simulink model "EKF"  (R2024b)
settings: Solver=ode4  StartTime=0.0  StopTime=10  FixedStep=1e-2  RelTol=1e-3
values from neighbouring files (symbols this model uses):
  L = 10e-2    (= 0.1)    [EKF.m]
  Q = eye(8)*0.1    [EKF.m]
  R = eye(2)*10    [EKF.m]
  r = 3.5e-2    (= 0.035)    [EKF.m]
  theta_0 = deg2rad(0)    [EKF.m]
  Ts = 1/10    (= 0.1)    [EKF.m]
libraries: simulink x5, sharedTrackingLibrary x1
settings Model: ParamWorkspaceSource=ReferencedWorkspace  Creator=pedro  LastModifiedBy=pedro
settings SFSimCC: SimCustomHeaderCode="#include \"EstimationSystem.h\""  SimUserSources=C:\Users\pedro\Documents\UNICAMP\embarcados\ekf_cross_plat\src\EstimationSystem.c  SimUserLibraries=C:\Users\pedro\Documents\UNICAMP\embarcados\ekf_cross_plat\build\lib\CMSIS-DSP\Source\libCMSISDSP.a  SimCustomCompilerFlags=-DARM_MATH_LOOPUNROLL -D__GNUC_PYTHON__  CustomCodeGlobalsAsFunctionIO=on  SimHardwareAcceleration=off
settings SFSimCC: SimUserIncludeDirs=|
  | C:\Users\pedro\Documents\UNICAMP\embarcados\ekf_cross_plat\inc
  | C:\Users\pedro\Documents\UNICAMP\embarcados\ekf_cross_plat\lib\CMSIS-DSP\Include
  | C:\Users\pedro\Documents\UNICAMP\embarcados\ekf_cross_plat\lib\CMSIS-DSP\PrivateInclude
  | C:\Users\pedro\Documents\UNICAMP\embarcados\ekf_cross_plat\lib\CMSIS-DSP\Source\DistanceFunctions
  | C:\Users\pedro\Documents\UNICAMP\embarcados\ekf_cross_plat\lib\CMSIS-DSP\ComputeLibrary
settings RTWCC: GenerateReport=on  RTWUseSimCustomCode=on  CustomHeaderCode="#include \"EstimationSystem.h\""  CustomSource=C:\Users\pedro\Documents\UNICAMP\embarcados\ekf_cross_plat\src\EstimationSystem.c  CustomLibrary=C:\Users\pedro\Documents\UNICAMP\embarcados\ekf_cross_plat\build\lib\CMSIS-DSP\Source\libCMSISDSP.a  BuildConfiguration=Debug  LaunchReport=on
settings RTWCC: CustomInclude=|
  | C:\Users\pedro\Documents\UNICAMP\embarcados\ekf_cross_plat\inc
  | C:\Users\pedro\Documents\UNICAMP\embarcados\ekf_cross_plat\lib\CMSIS-DSP\Include
  | C:\Users\pedro\Documents\UNICAMP\embarcados\ekf_cross_plat\lib\CMSIS-DSP\PrivateInclude
  | C:\Users\pedro\Documents\UNICAMP\embarcados\ekf_cross_plat\lib\CMSIS-DSP\Source\DistanceFunctions
  | C:\Users\pedro\Documents\UNICAMP\embarcados\ekf_cross_plat\lib\CMSIS-DSP\ComputeLibrary
settings CodeAppCC: MaxIdLength=95

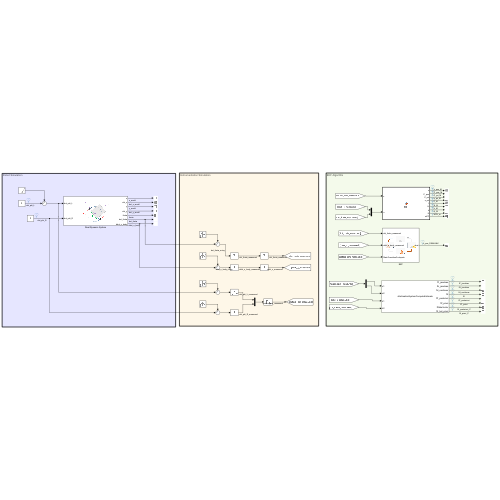
[thumbnail: Simulink's stored preview of the top-level diagram]
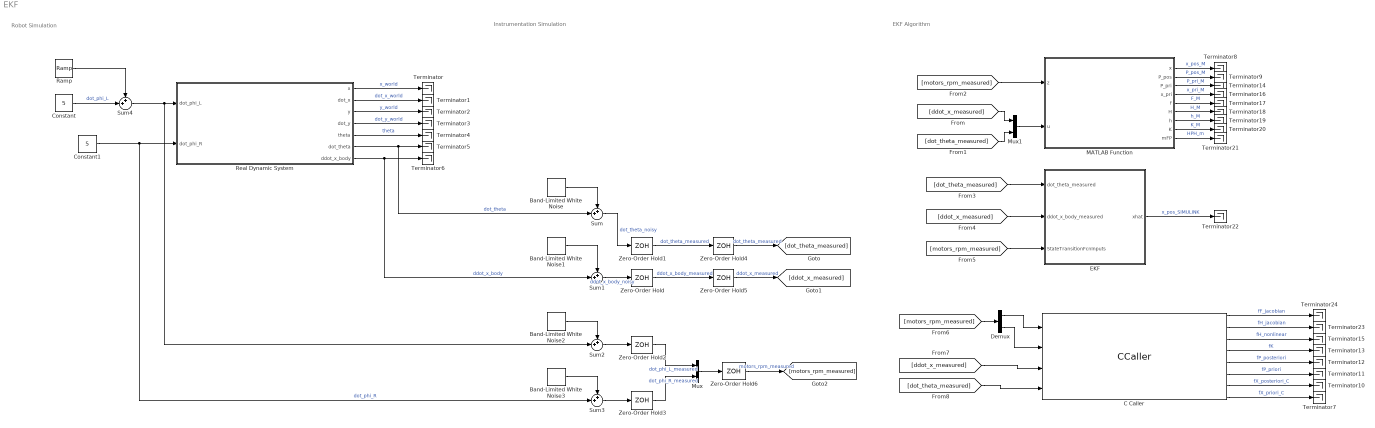
== system EKF ==
  note: EKF Algorithm
  note: Instrumentation Simulation
  note: Robot Simulation
  Band-Limited White Noise : simulink/Sources/Band-Limited White Noise  Cov=[0.0001]  Ts=0.1  seed=[23341]
  Band-Limited White Noise1 : simulink/Sources/Band-Limited White Noise  Cov=[0.0001]  Ts=0.1  seed=[23341]
  Band-Limited White Noise2 : simulink/Sources/Band-Limited White Noise  Cov=[0.001]  Ts=0.1  seed=[23341]
  Band-Limited White Noise3 : simulink/Sources/Band-Limited White Noise  Cov=[0.001]  Ts=0.1  seed=[23341]
  C Caller : CCaller  FunctionName=vEstimationSystemComputeEstimate  PortSpecificationStruct="%)30     .     !4   8    (     @         %    \"     P    !     0         %  0 \"0    $    _    07)G3F%M90  4&]R=$YA;64 4V-O<&4     26YD97@     5'EP90      4VEZ90      27-';&]B86P   X    P    !@    @    $          4    (     0    (    !         !   @!U,0  #@   #     &    \"     0         !0    @    !     @    $         $  \" '4Q   .    .     8    (    !          %    \"     $    %     0         0  ...(+6883 chars)"  SampleTime=Ts
  Constant : Constant  Value=5
  Constant1 : Constant  Value=5
  Demux : Demux  Outputs=2
  EKF : Subsystem
      mask Display: image('EKF_icon.png', [0,0,0,0,90,90]);
  MATLAB Function : MATLAB Function  TreatAsAtomicUnit=on
  Mux : Mux  Inputs=2
  Mux1 : Mux  Inputs=2
  Ramp : simulink/Sources/Ramp  slope=1  start=2  InitialOutput=0
  Real Dynamic System : Subsystem
      mask Display: image('robot_model.png', [0,0,0,0,90,90]);
  Sum{,1..4} (5 alike) : Sum  Inputs=++|
  Terminator{,1..24} (25 alike) : Terminator
  Zero-Order Hold{,1..6} (7 alike) : ZeroOrderHold  SampleTime=Ts
  wires:
  Constant/1 -> Sum4/2  "dot_phi_L"
  Constant1/1 -> Real Dynamic System/2(dot_phi_R), Sum3/2  "dot_phi_R"
  Real Dynamic System/1(x) -> Terminator/1  "x_world"
  Real Dynamic System/2(dot_x) -> Terminator1/1  "dot_x_world"
  Real Dynamic System/3(y) -> Terminator2/1  "y_world"
  Real Dynamic System/4(dot_y) -> Terminator3/1  "dot_y_world"
  Real Dynamic System/5(theta) -> Terminator4/1  "theta"
  Real Dynamic System/6(dot_theta) -> Sum/2, Terminator5/1  "dot_theta"
  Real Dynamic System/7(ddot_x_body) -> Sum1/2, Terminator6/1  "ddot_x_body"
  Band-Limited White Noise/1 -> Sum/1
  Sum/1 -> Zero-Order Hold1/1  "dot_theta_noisy"
  Band-Limited White Noise1/1 -> Sum1/1
  Sum1/1 -> Zero-Order Hold/1  "ddot_x_body_noisy"
  Band-Limited White Noise2/1 -> Sum2/1
  Band-Limited White Noise3/1 -> Sum3/1
  Sum2/1 -> Zero-Order Hold2/1
  Sum3/1 -> Zero-Order Hold3/1
  Mux/1 -> Zero-Order Hold6/1
  Zero-Order Hold1/1 -> Zero-Order Hold4/1  "dot_theta_measured"
  Zero-Order Hold/1 -> Zero-Order Hold5/1  "ddot_x_body_measured"
  Zero-Order Hold2/1 -> Mux/1  "dot_phi_L_measured"
  Zero-Order Hold3/1 -> Mux/2  "dot_phi_R_measured"
  Zero-Order Hold4/1 -> [dot_theta_measured]  "dot_theta_measured"
  Zero-Order Hold5/1 -> [ddot_x_measured]  "ddot_x_measured"
  Zero-Order Hold6/1 -> [motors_rpm_measured]  "motors_rpm_measured"
  Sum4/1 -> Sum2/2, Real Dynamic System/1(dot_phi_L)
  Ramp/1 -> Sum4/1
  MATLAB Function/1(x) -> Terminator8/1  "x_pos_M"
  [ddot_x_measured] -> Mux1/1
  [dot_theta_measured] -> Mux1/2
  [dot_theta_measured] -> EKF/1(dot_theta_measured)
  [ddot_x_measured] -> EKF/2(ddot_x_body_measured)
  [motors_rpm_measured] -> EKF/3(StateTransitionFcnInputs)
  [motors_rpm_measured] -> Demux/1
  Demux/1 -> C Caller/1
  Demux/2 -> C Caller/2
  [ddot_x_measured] -> C Caller/3
  [dot_theta_measured] -> C Caller/4
  Mux1/1 -> MATLAB Function/2(u)
  [motors_rpm_measured] -> MATLAB Function/1(z)
  MATLAB Function/2(P_pos) -> Terminator9/1  "P_pos_M"
  MATLAB Function/3(P_pri) -> Terminator14/1  "P_pri_M"
  MATLAB Function/4(x_pri) -> Terminator16/1  "x_pri_M"
  MATLAB Function/5(f) -> Terminator17/1  "F_M"
  MATLAB Function/6(H) -> Terminator18/1  "H_M"
  MATLAB Function/7(h) -> Terminator19/1  "h_M"
  MATLAB Function/8(K) -> Terminator20/1  "K_M"
  MATLAB Function/9(mFP) -> Terminator21/1  "HPH_m"
  EKF/1(xhat) -> Terminator22/1  "x_pos_SIMULINK"
  C Caller/8 -> Terminator7/1  "fX_priori_C"
  C Caller/7 -> Terminator10/1  "fX_posteriori_C"
  C Caller/6 -> Terminator11/1  "fP_priori"
  C Caller/5 -> Terminator12/1  "fP_posteriori"
  C Caller/4 -> Terminator13/1  "fK"
  C Caller/3 -> Terminator15/1  "fH_nonlinear"
  C Caller/2 -> Terminator23/1  "fH_jacobian"
  C Caller/1 -> Terminator24/1  "fF_jacobian"

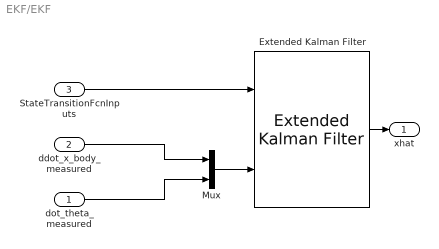
== system EKF/EKF ==
  dot_theta_measured : Inport
  ddot_x_body_measured : Inport  Port=2
  StateTransitionFcnInputs : Inport  Port=3
  Extended Kalman Filter : sharedTrackingLibrary/Extended Kalman Filter  StateTransitionFcn=DifferentialRobotModel  HasStateTransitionJacobianFcn=on  StateTransitionJacobianFcn=A_Jacobian  HasAdditiveProcessNoise=Additive  ProcessNoise=eye(8)*0.1  HasTimeVaryingProcessNoise=off  HasStateTransitionFcnExtraArgument=1  InitialState=states_0  InitialStateCovariance=eye(8)*0.1  MeasurementFcn1=OBSERVATION_h  HasMeasurementJacobianFcn1=on  MeasurementJacobianFcn1=H_jacobian  HasMeasurementEnablePort1=off  HasAdditiveMeasurementNoise1=Additive  MeasurementNoise1=eye(2)*10  HasTimeVaryingMeasurementNoise1=off  HasMeasurementFcnExtraArgument1=0  HasMeasurementWrapping1=off  MeasurementFcn2=OBSERVATION_x_ddot_body  HasMeasurementJacobianFcn2=off  HasMeasurementEnablePort2=off  HasAdditiveMeasurementNoise2=Additive  MeasurementNoise2=0.1  HasTimeVaryingMeasurementNoise2=off  HasMeasurementFcnExtraArgument2=0  HasMeasurementWrapping2=off  MeasurementFcn3=myMeasurementFcn  HasMeasurementJacobianFcn3=off  HasMeasurementEnablePort3=off  HasAdditiveMeasurementNoise3=Additive  MeasurementNoise3=1  HasTimeVaryingMeasurementNoise3=off  HasMeasurementFcnExtraArgument3=0  HasMeasurementWrapping3=off  MeasurementFcn4=myMeasurementFcn  HasMeasurementJacobianFcn4=off  HasMeasurementEnablePort4=off  HasAdditiveMeasurementNoise4=Additive  MeasurementNoise4=1  HasTimeVaryingMeasurementNoise4=off  HasMeasurementFcnExtraArgument4=0  HasMeasurementWrapping4=off  MeasurementFcn5=myMeasurementFcn  HasMeasurementJacobianFcn5=off  HasMeasurementEnablePort5=off  HasAdditiveMeasurementNoise5=Additive  MeasurementNoise5=1  HasTimeVaryingMeasurementNoise5=off  HasMeasurementFcnExtraArgument5=0  HasMeasurementWrapping5=off  EnableMultirate=off  StateTransitionFcnSampleTime=1  MeasurementFcn1SampleTime=1  MeasurementFcn2SampleTime=1  MeasurementFcn3SampleTime=1  MeasurementFcn4SampleTime=1  MeasurementFcn5SampleTime=1  UseCurrentEstimator=on  OutputStateCovariance=off  DataType=double  SampleTime=Ts  NumberOfMeasurements=1
  Mux : Mux  Inputs=2
  xhat : Outport
  wires:
  Extended Kalman Filter/1 -> xhat/1
  StateTransitionFcnInputs/1 -> Extended Kalman Filter/1
  Mux/1 -> Extended Kalman Filter/2
  dot_theta_measured/1 -> Mux/2
  ddot_x_body_measured/1 -> Mux/1

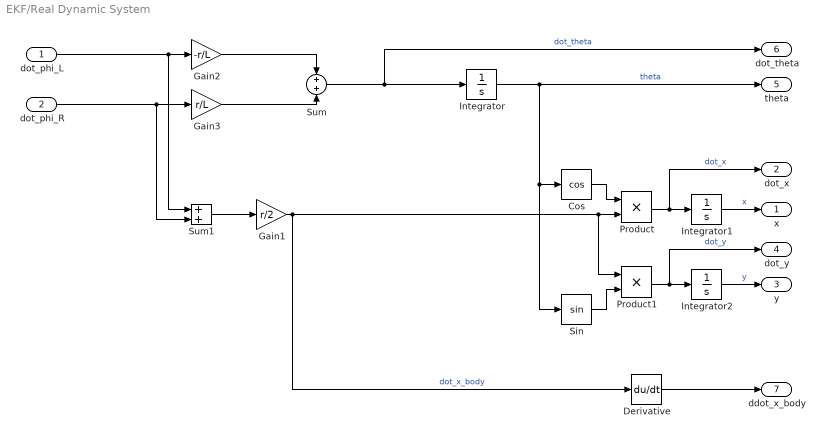
== system EKF/Real Dynamic System ==
  dot_phi_L : Inport
  dot_phi_R : Inport  Port=2
  Cos : Trigonometry  Operator=cos
  Derivative : Derivative
  Gain1 : Gain  Gain=r/2
  Gain2 : Gain  Gain=-r/L
  Gain3 : Gain  Gain=r/L
  Integrator : Integrator  InitialCondition=theta_0
  Integrator1 : Integrator
  Integrator2 : Integrator
  Product : Product
  Product1 : Product
  Sin : Trigonometry
  Sum : Sum  Inputs=+|+
  Sum1 : Sum
  x : Outport
  dot_x : Outport  Port=2
  y : Outport  Port=3
  dot_y : Outport  Port=4
  theta : Outport  Port=5
  dot_theta : Outport  Port=6
  ddot_x_body : Outport  Port=7
  wires:
  dot_phi_L/1 -> Sum1/1, Gain2/1
  Product1/1 -> dot_y/1, Integrator2/1  "dot_y"
  Cos/1 -> Product/1
  Integrator/1 -> theta/1, Sin/1, Cos/1  "theta"
  Gain3/1 -> Sum/2
  Product/1 -> dot_x/1, Integrator1/1  "dot_x"
  Gain1/1 -> Derivative/1, Product1/1, Product/2  "dot_x_body"
  Sum1/1 -> Gain1/1
  dot_phi_R/1 -> Sum1/2, Gain3/1
  Gain2/1 -> Sum/1
  Sum/1 -> dot_theta/1, Integrator/1  "dot_theta"
  Integrator1/1 -> x/1  "x"
  Integrator2/1 -> y/1  "y"
  Sin/1 -> Product1/2
  Derivative/1 -> ddot_x_body/1

== matlab function EKF/MATLAB Function ==
  data: z input; u input; x output; P_pos output; P_pri output; x_pri output; R parameter; Q parameter; f output; H output size=[2 8]; h output size=[2 1]; K output; mFP output
function [x, P_pos, P_pri, x_pri, f, H, h, K, mFP] = fcn(z,u, R, Q)

[x, P_pos, P_pri, x_pri, f, H, h, K, mFP] = EKF_algo(z, u, R, Q);
